simulink model "exerc_3"  (R2018b)
settings: Solver=VariableStepAuto  StartTime=0.0  StopTime=30  RelTol=1e-3
values from neighbouring files (symbols this model uses):
  A = [   -1,    1,    2,    2.5 ... (first row only)    [exercicio_01.m]    (also in exercicio_03.m = [-2.068, -2; 2, 0]; exercicio_03_2.m = [-2.068, -2; 2, 0])
  B = [1; 0]    [exercicio_03.m]    (also in exercicio_03_2.m)
  C = [1, -0.4]    [exercicio_03.m]    (also in exercicio_03_2.m)
  D = 0    [exercicio_03.m]    (also in exercicio_03_2.m)
  uop = 30    [exercicio_03.m]    (also in exercicio_03_2.m)
  yop = 20    [exercicio_03.m]    (also in exercicio_03_2.m)
settings Model: Creator=bernardo  LastModifiedBy=bernardo

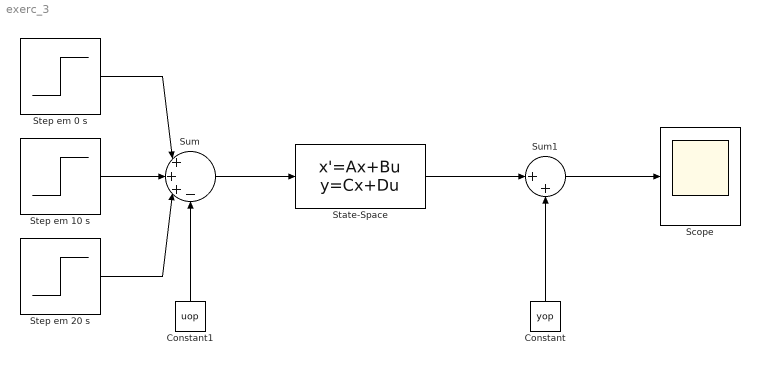
== system exerc_3 ==
  Constant : Constant  Value=yop
  Constant1 : Constant  Value=uop
  Scope : Scope
  State-Space : StateSpace  A=A  B=B  C=[C]  D=[D]  InitialCondition=0
  "Step em 0 s " : Step  Time=0  Before=30  After=35  SampleTime=0.001
  Step em 10 s : Step  Time=10  After=-10  SampleTime=0.001
  Step em 20 s : Step  Time=20  After=5  SampleTime=0.001
  Sum : Sum  Inputs=|+++-
  Sum1 : Sum  Inputs=|++
  wires:
  Step em 10 s/1 -> Sum/2
  "Step em 0 s "/1 -> Sum/1
  Step em 20 s/1 -> Sum/3
  Sum/1 -> State-Space/1
  Sum1/1 -> Scope/1
  Constant/1 -> Sum1/2
  Constant1/1 -> Sum/4
  State-Space/1 -> Sum1/1
